simulink model "gm_sampleModel1471_5_sub"  (R2023a)
settings: Solver=VariableStepAuto  StartTime=0.0  StopTime=10.0  RelTol=1e-3
libraries: simulink x5, hdlsllib x1
settings Model: Creator=user1  LastModifiedBy=user1
settings OptimizationCC: BlockReduction=off  ConditionallyExecuteInputs=off
settings DebuggingCC: InheritedTsInSrcMsg=none

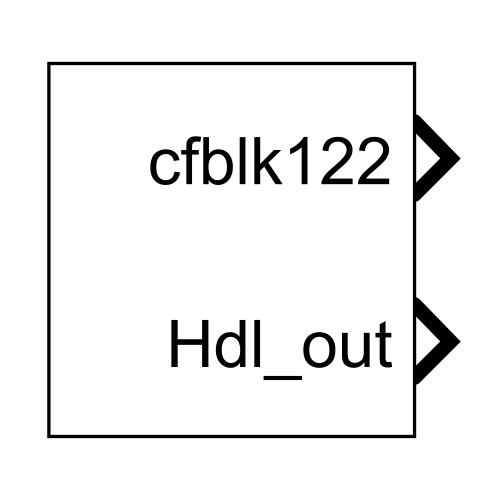
[thumbnail: Simulink's stored preview of the top-level diagram]
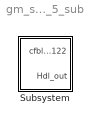
== system gm_sampleModel1471_5_sub ==
  Subsystem : Subsystem

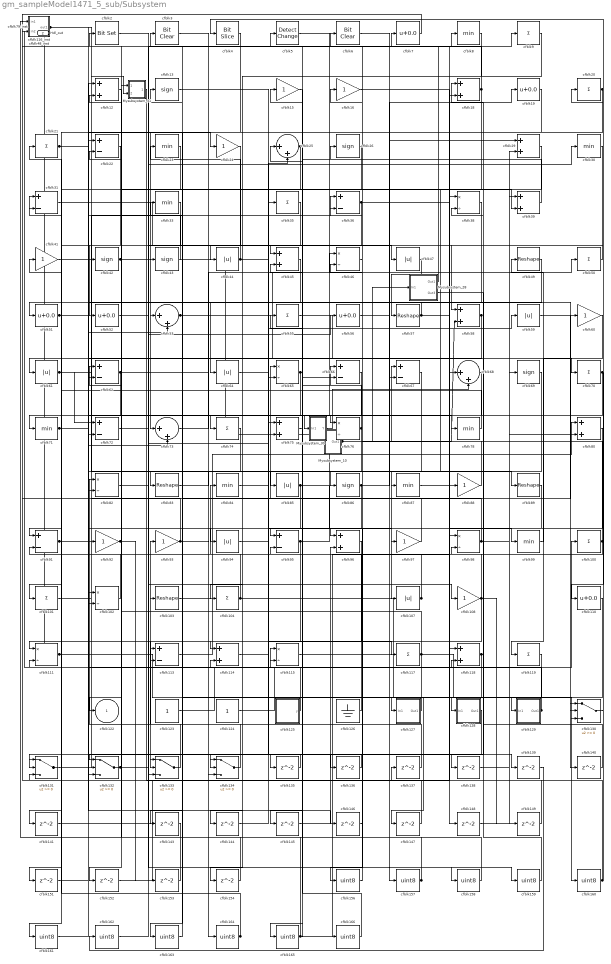
== system gm_sampleModel1471_5_sub/Subsystem ==
  Mysubsystem_10 : Subsystem
  Mysubsystem_28 : Subsystem
  Mysubsystem_30 : Subsystem
  Mysubsystem_31 : Subsystem
  cfblk{9,20..21,35,50,55,70,74,100..101,104,117,119} (13 alike) : Sum  Inputs=+  OutDataTypeStr=uint8
  cfblk{38,46,65,76,82,98,102,111,115} (9 alike) : Product  Inputs=*/  OutDataTypeStr=uint8  RndMeth=Zero  SaturateOnIntegerOverflow=on
  cfblk{49,57,83,89,103} (5 alike) : Reshape
  cfblk{44,47,59,61,64,85,94,107} (8 alike) : Abs  OutDataTypeStr=uint8  SaturateOnIntegerOverflow=off
  cfblk{15..16,24,41,60,88,92..93,97,108} (10 alike) : Gain  OutDataTypeStr=uint8
  cfblk{7,19,51..52,56,110} (6 alike) : Bias  Bias=0.0  SaturateOnIntegerOverflow=off
  cfblk{22,31,36,62,66..67,72,91,95,113} (10 alike) : Sum  Inputs=+-  OutDataTypeStr=uint8
  cfblk{12,18,29,39,45,58,75,80,96,114,118} (11 alike) : Sum  OutDataTypeStr=uint8
  cfblk116_inst : Subsystem
  cfblk123 : Constant  OutDataTypeStr=uint8  SampleTime=-1
  cfblk124 : Constant  OutDataTypeStr=uint8  SampleTime=-1
  cfblk125 : Subsystem  mask(Counter Free-Running){NumBits=double(16), tsamp=double(-1)}
      mask prompts: NumBits "Simulink:masks:NumberOfBits_MP"; tsamp "Simulink:masks:SampleTime_MP"
      mask help: Simulink:masks:CounterFreeRunning_MD
  cfblk126 : Ground
  cfblk127 : Subsystem
  cfblk128 : Subsystem
  cfblk129 : Subsystem
  cfblk{13,26,42..43,69,86} (6 alike) : Signum
  cfblk{130..134} (5 alike) : Switch  OutDataTypeStr=uint8  SaturateOnIntegerOverflow=off  InputSameDT=off
  cfblk{135..141,143..149,151..154} (18 alike) : Delay  SampleTime=1
  cfblk{156..166} (11 alike) : DataTypeConversion  OutDataTypeStr=uint8  SaturateOnIntegerOverflow=off  RndMeth=Floor
  cfblk2 : simulink/Logic and Bit Operations/Bit Set  iBit=0
      settings: LibrarySourceBlock=|
      | hdlsllib/Logic and Bit
      | Operations/Bit Set
  cfblk{8,23,30,33,71,78,84,87,99} (9 alike) : MinMax  OutDataTypeStr=uint8
  cfblk{25,53,68,73} (4 alike) : Sum  Inputs=|++  OutDataTypeStr=uint8
  cfblk3 : simulink/Logic and Bit Operations/Bit Clear  iBit=0
      settings: LibrarySourceBlock=|
      | hdlsllib/Logic and Bit
      | Operations/Bit Clear
  cfblk4 : hdlsllib/Logic and Bit Operations/Bit Slice  lidx=7  ridx=0
  cfblk48_inst : Subsystem
  cfblk5 : simulink/Logic and Bit Operations/Detect Change  vinit=0  OutDataTypeStr=uint8
      settings: LibrarySourceBlock=|
      | hdlsllib/Logic and Bit
      | Operations/Detect
      | Change
  cfblk6 : simulink/Logic and Bit Operations/Bit Clear  iBit=0
      settings: LibrarySourceBlock=|
      | hdlsllib/Logic and Bit
      | Operations/Bit Clear
  cfblk79_inst : Subsystem
  cfblk122 : Outport  OutDataTypeStr=uint8  SampleTime=1  VectorParamsAs1DForOutWhenUnconnected=off
  Hdl_out : Outport  Port=2  OutDataTypeStr=uint8  SampleTime=1
  wires:
  Mysubsystem_10/1(Out1) -> cfblk58/2, Mysubsystem_28/1(In1)
  Mysubsystem_28/1(Out1) -> cfblk7/1
  Mysubsystem_28/2(Out3) -> cfblk133/2
  Mysubsystem_30/1(Y) -> cfblk68/2
  Mysubsystem_31/1(Out1) -> cfblk137/1
  cfblk100/1 -> cfblk91/2, cfblk67/1
  cfblk101/1 -> cfblk36/1
  cfblk102/1 -> cfblk82/1
  cfblk103/1 -> cfblk80/1
  cfblk104/1 -> cfblk128/1(In1), cfblk84/1
  cfblk107/1 -> cfblk95/2, cfblk26/1
  cfblk108/1 -> cfblk36/2, cfblk133/1, cfblk149/1
  cfblk110/1 -> cfblk127/1(In1)
  cfblk111/1 -> Hdl_out/1, cfblk129/1(In1)
  cfblk113/1 -> cfblk65/1
  cfblk114/1 -> cfblk35/1
  cfblk115/1 -> cfblk160/1
  cfblk116_inst/1(out1) -> cfblk107/1, Mysubsystem_31/2(In2)
  cfblk117/1 -> cfblk22/2, cfblk130/3, cfblk114/2
  cfblk118/1 -> cfblk18/1, cfblk147/1
  cfblk119/1 -> cfblk163/1
  cfblk12/1 -> cfblk39/2
  cfblk123/1 -> cfblk18/2
  cfblk124/1 -> cfblk100/1
  cfblk125/1(y) -> cfblk62/1
  cfblk126/1 -> cfblk12/2
  cfblk127/1(Out1) -> cfblk46/2
  cfblk128/1(Out1) -> cfblk135/1
  cfblk129/1(Out1) -> cfblk79_inst/2(in2), cfblk45/2, cfblk25/1
  cfblk13/1 -> cfblk75/2
  cfblk130/1 -> cfblk4/1
  cfblk131/1 -> cfblk60/1
  cfblk132/1 -> cfblk75/1, cfblk8/1
  cfblk133/1 -> cfblk92/1
  cfblk134/1 -> cfblk93/1
  cfblk135/1 -> cfblk131/2
  cfblk136/1 -> cfblk134/2
  cfblk137/1 -> cfblk102/1
  cfblk138/1 -> cfblk39/1
  cfblk139/1 -> cfblk162/1
  cfblk140/1 -> cfblk118/2
  cfblk141/1 -> cfblk68/1
  cfblk143/1 -> cfblk116_inst/1(in1)
  cfblk144/1 -> cfblk65/2
  cfblk145/1 -> cfblk96/2
  cfblk146/1 -> cfblk66/1
  cfblk147/1 -> cfblk131/3
  cfblk148/1 -> cfblk80/2
  cfblk149/1 -> cfblk113/2
  cfblk15/1 -> cfblk165/1
  cfblk151/1 -> cfblk82/2
  cfblk152/1 -> cfblk25/2
  cfblk153/1 -> cfblk111/2
  cfblk154/1 -> cfblk22/1
  cfblk156/1 -> cfblk6/1
  cfblk157/1 -> cfblk31/1, cfblk41/1
  cfblk158/1 -> cfblk2/1
  cfblk159/1 -> cfblk98/2
  cfblk16/1 -> cfblk99/1
  cfblk160/1 -> cfblk48_inst/2(in2), cfblk38/2, cfblk20/1
  cfblk161/1 -> cfblk115/1
  cfblk162/1 -> cfblk115/2
  cfblk163/1 -> cfblk3/1
  cfblk164/1 -> cfblk31/2, cfblk103/1
  cfblk165/1 -> cfblk13/1, cfblk98/1
  cfblk166/1 -> cfblk15/1
  cfblk18/1 -> cfblk79_inst/1(in1), cfblk134/3
  cfblk19/1 -> cfblk143/1
  cfblk2/1 -> cfblk159/1
  cfblk20/1 -> cfblk73/1, cfblk51/1
  cfblk21/1 -> cfblk67/2, cfblk53/1
  cfblk22/1 -> cfblk91/1
  cfblk23/1 -> cfblk132/1
  cfblk24/1 -> cfblk132/3
  cfblk25/1 -> cfblk61/1, cfblk131/1
  cfblk26/1 -> cfblk145/1
  cfblk29/1 -> cfblk87/1
  cfblk3/1 -> cfblk164/1
  cfblk30/1 -> cfblk58/1
  cfblk31/1 -> cfblk47/1
  cfblk33/1 -> cfblk52/1
  cfblk35/1 -> cfblk83/1
  cfblk36/1 -> cfblk148/1, cfblk104/1
  cfblk38/1 -> cfblk144/1
  cfblk39/1 -> cfblk5/1
  cfblk4/1 -> cfblk43/1
  cfblk41/1 -> cfblk130/2
  cfblk42/1 -> cfblk44/1, cfblk76/2
  cfblk43/1 -> cfblk12/1
  cfblk44/1 -> cfblk96/1, cfblk23/1
  cfblk45/1 -> cfblk64/1
  cfblk46/1 -> cfblk16/1
  cfblk47/1 -> cfblk57/1
  cfblk48_inst/1(out1) -> cfblk53/2
  cfblk49/1 -> cfblk141/1
  cfblk5/1 -> cfblk118/1
  cfblk50/1 -> cfblk45/1
  cfblk51/1 -> cfblk139/1, cfblk78/1
  cfblk52/1 -> cfblk30/1
  cfblk53/1 -> cfblk29/2, cfblk140/1
  cfblk55/1 -> cfblk70/1
  cfblk56/1 -> cfblk158/1
  cfblk57/1 -> Mysubsystem_31/1(In1), cfblk9/1
  cfblk58/1 -> cfblk151/1, cfblk101/1
  cfblk59/1 -> cfblk130/1
  cfblk6/1 -> cfblk157/1
  cfblk60/1 -> cfblk119/1
  cfblk61/1 -> cfblk89/1, cfblk72/1
  cfblk62/1 -> cfblk72/2, Mysubsystem_30/1(In1)
  cfblk64/1 -> cfblk138/1
  cfblk65/1 -> cfblk94/1, cfblk166/1
  cfblk66/1 -> cfblk71/1
  cfblk67/1 -> cfblk114/1
  cfblk68/1 -> cfblk85/1
  cfblk69/1 -> cfblk152/1
  cfblk7/1 -> cfblk48_inst/1(in1)
  cfblk70/1 -> cfblk110/1, cfblk74/1
  cfblk71/1 -> cfblk73/2, cfblk146/1
  cfblk72/1 -> cfblk56/1
  cfblk73/1 -> cfblk50/1
  cfblk74/1 -> cfblk132/2
  cfblk75/1 -> cfblk66/2
  cfblk76/1 -> cfblk95/1, cfblk55/1
  cfblk78/1 -> cfblk21/1
  cfblk79_inst/1(out1) -> cfblk24/1
  cfblk8/1 -> cfblk134/1
  cfblk80/1 -> cfblk102/2
  cfblk82/1 -> cfblk108/1
  cfblk83/1 -> cfblk86/1
  cfblk84/1 -> cfblk59/1
  cfblk85/1 -> cfblk113/1, cfblk97/1
  cfblk86/1 -> cfblk29/1, cfblk19/1, cfblk122/1
  cfblk87/1 -> cfblk88/1
  cfblk88/1 -> cfblk46/1
  cfblk89/1 -> cfblk156/1
  cfblk9/1 -> cfblk154/1
  cfblk91/1 -> cfblk42/1, cfblk133/3
  cfblk92/1 -> cfblk62/2, cfblk153/1
  cfblk93/1 -> cfblk116_inst/2(in2), cfblk136/1
  cfblk94/1 -> cfblk117/1
  cfblk95/1 -> cfblk161/1, cfblk38/1
  cfblk96/1 -> cfblk111/1
  cfblk97/1 -> cfblk76/1
  cfblk98/1 -> cfblk69/1, cfblk33/1
  cfblk99/1 -> cfblk49/1

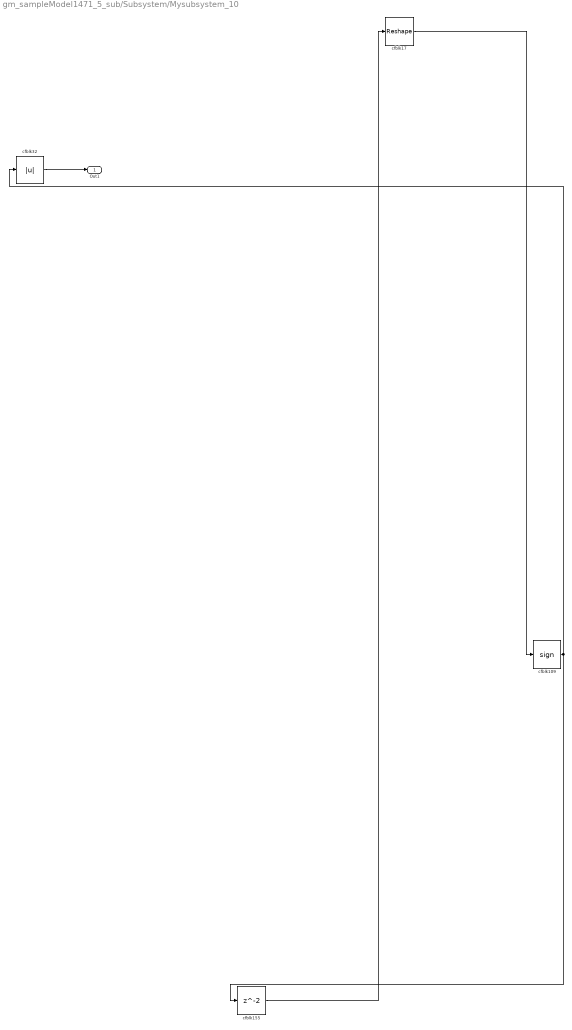
== system gm_sampleModel1471_5_sub/Subsystem/Mysubsystem_10 ==
  cfblk109 : Signum
  cfblk155 : Delay  SampleTime=1
  cfblk17 : Reshape
  cfblk32 : Abs  SaturateOnIntegerOverflow=off
  Out1 : Outport  SampleTime=1
  wires:
  cfblk109/1 -> cfblk32/1, cfblk155/1
  cfblk155/1 -> cfblk17/1
  cfblk17/1 -> cfblk109/1
  cfblk32/1 -> Out1/1

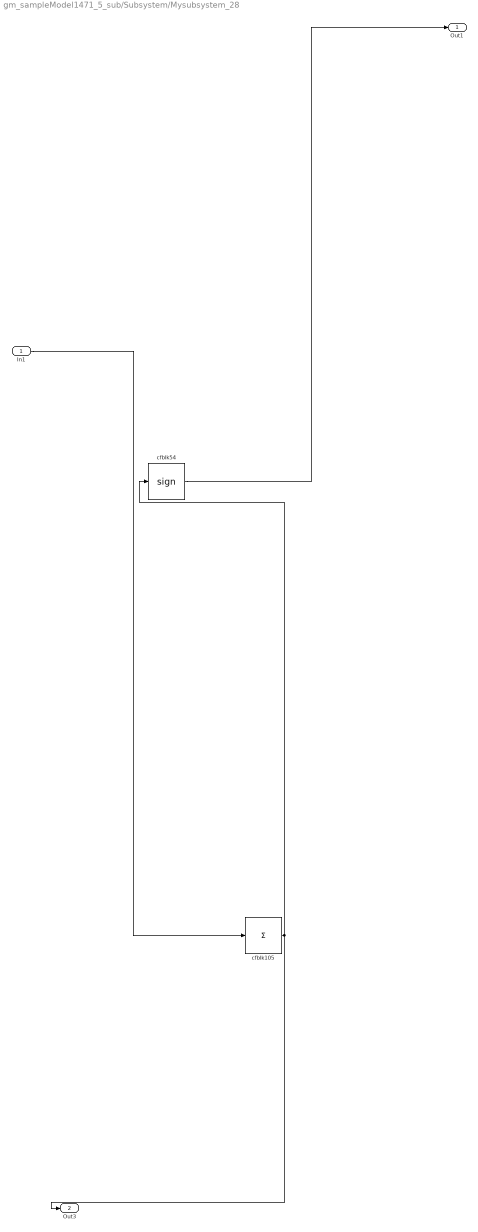
== system gm_sampleModel1471_5_sub/Subsystem/Mysubsystem_28 ==
  In1 : Inport  OutDataTypeStr=uint8  PortDimensions=1  SampleTime=1
  cfblk105 : Sum  Inputs=+
  cfblk54 : Signum
  Out1 : Outport  SampleTime=1
  Out3 : Outport  Port=2  SampleTime=1
  wires:
  In1/1 -> cfblk105/1
  cfblk105/1 -> cfblk54/1, Out3/1
  cfblk54/1 -> Out1/1

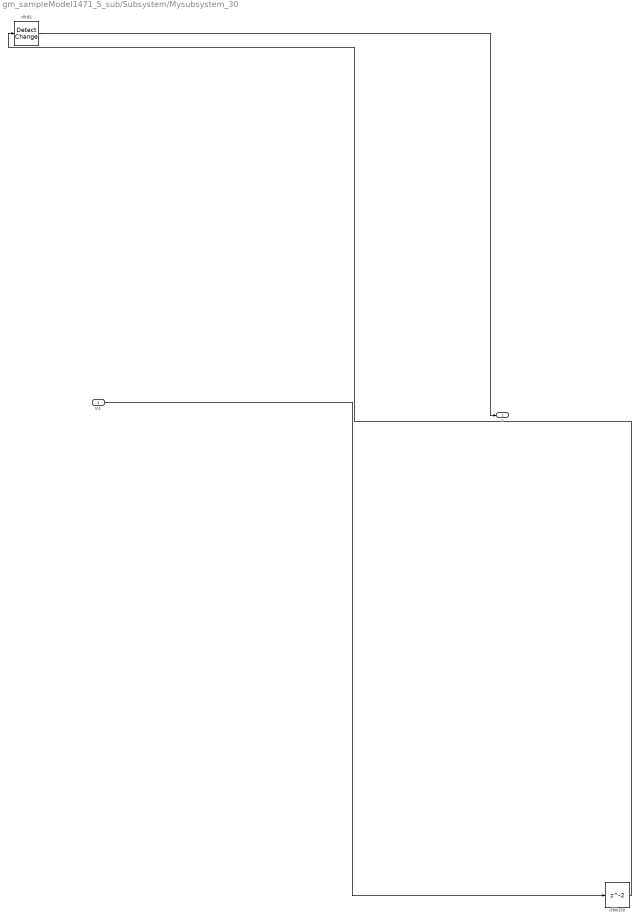
== system gm_sampleModel1471_5_sub/Subsystem/Mysubsystem_30 ==
  In1 : Inport  OutDataTypeStr=uint8  PortDimensions=1  SampleTime=1
  cfblk1 : simulink/Logic and Bit Operations/Detect Change  vinit=0  OutDataTypeStr=boolean
      settings: LibrarySourceBlock=|
      | hdlsllib/Logic and Bit
      | Operations/Detect
      | Change
  cfblk150 : Delay  SampleTime=1
  Y : Outport  SampleTime=1
  wires:
  In1/1 -> cfblk150/1
  cfblk1/1 -> Y/1
  cfblk150/1 -> cfblk1/1

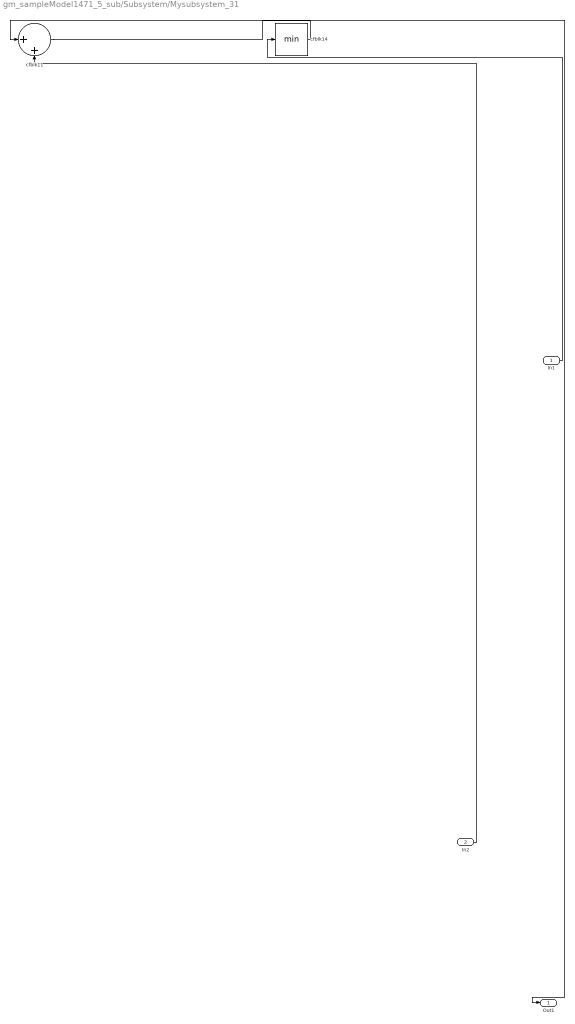
== system gm_sampleModel1471_5_sub/Subsystem/Mysubsystem_31 ==
  In1 : Inport  OutDataTypeStr=uint8  PortDimensions=1  SampleTime=1
  In2 : Inport  Port=2  OutDataTypeStr=uint8  PortDimensions=1  SampleTime=1
  cfblk11 : Sum  Inputs=|++
  cfblk14 : MinMax
  Out1 : Outport  SampleTime=1
  wires:
  In1/1 -> cfblk14/1
  In2/1 -> cfblk11/2
  cfblk11/1 -> Out1/1
  cfblk14/1 -> cfblk11/1

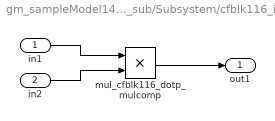
== system gm_sampleModel1471_5_sub/Subsystem/cfblk116_inst ==
  in1 : Inport  OutDataTypeStr=uint8  SampleTime=1
  in2 : Inport  Port=2  OutDataTypeStr=uint8  SampleTime=1
  mul_cfblk116_dotp_mulcomp : Product  Inputs=**  OutDataTypeStr=uint8  SampleTime=1
  out1 : Outport  OutDataTypeStr=uint8  SampleTime=1
  wires:
  in1/1 -> mul_cfblk116_dotp_mulcomp/1
  in2/1 -> mul_cfblk116_dotp_mulcomp/2
  mul_cfblk116_dotp_mulcomp/1 -> out1/1

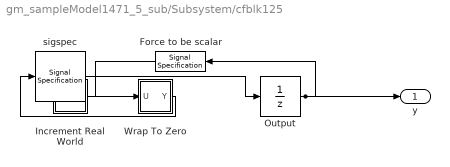
== system gm_sampleModel1471_5_sub/Subsystem/cfblk125 ==
  Force to be scalar : SignalSpecification  DisableCoverage=on  Dimensions=1
  Increment Real World : Subsystem  mask(Real World Value Increment){}
      mask help: Simulink:masks:RealWorldValueIncrement_MD
      mask Display: disp('V++')
  Output : UnitDelay  InitialCondition=0.0  SampleTime=tsamp  HasFrameUpgradeWarning=on
  Wrap To Zero : Subsystem  mask(Wrap To Zero){Threshold=double(65535)}
      mask prompts: Threshold "Simulink:masks:Threshold_MP"
      mask help: Simulink:masks:WrapToZero_MD
  sigspec : SignalSpecification  OutDataTypeStr=uint16  Dimensions=1
  y : Outport  SampleTime=1
  wires:
  Force to be scalar/1 -> Increment Real World/1(u)
  Increment Real World/1(y) -> Wrap To Zero/1(U)
  Output/1 -> Force to be scalar/1, y/1
  Wrap To Zero/1(Y) -> sigspec/1
  sigspec/1 -> Output/1

== system gm_sampleModel1471_5_sub/Subsystem/cfblk127 ==
  In1 : Inport  OutDataTypeStr=uint8  PortDimensions=1  SampleTime=1
  Out1 : Outport  SampleTime=1
  wires:
  In1/1 -> Out1/1

== system gm_sampleModel1471_5_sub/Subsystem/cfblk128 ==
  In1 : Inport  OutDataTypeStr=uint8  PortDimensions=1  SampleTime=1
  Out1 : Outport  SampleTime=1
  wires:
  In1/1 -> Out1/1

== system gm_sampleModel1471_5_sub/Subsystem/cfblk129 ==
  In1 : Inport  OutDataTypeStr=uint8  PortDimensions=1  SampleTime=1
  Out1 : Outport  SampleTime=1
  wires:
  In1/1 -> Out1/1

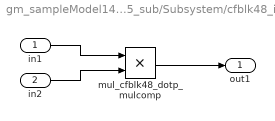
== system gm_sampleModel1471_5_sub/Subsystem/cfblk48_inst ==
  in1 : Inport  OutDataTypeStr=uint8  SampleTime=1
  in2 : Inport  Port=2  OutDataTypeStr=uint8  SampleTime=1
  mul_cfblk48_dotp_mulcomp : Product  Inputs=**  OutDataTypeStr=uint8  SampleTime=1
  out1 : Outport  OutDataTypeStr=uint8  SampleTime=1
  wires:
  in1/1 -> mul_cfblk48_dotp_mulcomp/1
  in2/1 -> mul_cfblk48_dotp_mulcomp/2
  mul_cfblk48_dotp_mulcomp/1 -> out1/1

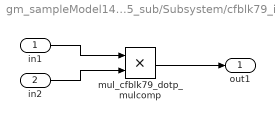
== system gm_sampleModel1471_5_sub/Subsystem/cfblk79_inst ==
  in1 : Inport  OutDataTypeStr=uint8  SampleTime=1
  in2 : Inport  Port=2  OutDataTypeStr=uint8  SampleTime=1
  mul_cfblk79_dotp_mulcomp : Product  Inputs=**  OutDataTypeStr=uint8  SampleTime=1
  out1 : Outport  OutDataTypeStr=uint8  SampleTime=1
  wires:
  in1/1 -> mul_cfblk79_dotp_mulcomp/1
  in2/1 -> mul_cfblk79_dotp_mulcomp/2
  mul_cfblk79_dotp_mulcomp/1 -> out1/1

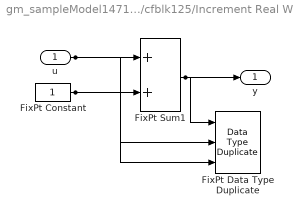
== system gm_sampleModel1471_5_sub/Subsystem/cfblk125/Increment Real World ==
  u : Inport  OutDataTypeStr=uint16  SampleTime=1
  FixPt Constant : Constant  DisableCoverage=on  OutDataTypeStr=Inherit: Inherit via back propagation  SampleTime=-1
  FixPt Data Type Duplicate : DataTypeDuplicate  DisableCoverage=on  NumInputPorts=3
  FixPt Sum1 : Sum  InputSameDT=on  OutDataTypeStr=Inherit: Inherit via back propagation  LockScale=on
  y : Outport  SampleTime=1
  wires:
  u/1 -> FixPt Sum1/1, FixPt Data Type Duplicate/2
  FixPt Constant/1 -> FixPt Sum1/2, FixPt Data Type Duplicate/3
  FixPt Sum1/1 -> FixPt Data Type Duplicate/1, y/1

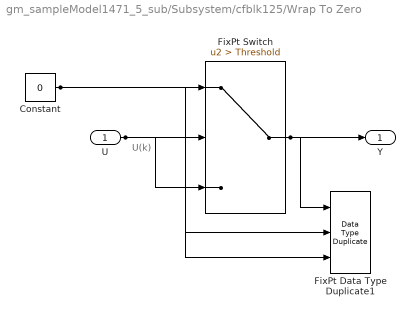
== system gm_sampleModel1471_5_sub/Subsystem/cfblk125/Wrap To Zero ==
  note: U(k)
  U : Inport  OutDataTypeStr=uint16  SampleTime=1
  Constant : Constant  DisableCoverage=on  Value=0  OutDataTypeStr=Inherit: Inherit via back propagation  SampleTime=-1
  FixPt Data Type Duplicate1 : DataTypeDuplicate  DisableCoverage=on  NumInputPorts=3
  FixPt Switch : Switch  Criteria=u2 > Threshold  Threshold=Threshold  OutDataTypeStr=Inherit: Inherit via back propagation  ZeroCross=off  SaturateOnIntegerOverflow=off  InputSameDT=off
  Y : Outport  SampleTime=1
  wires:
  U/1 -> FixPt Switch/3, FixPt Switch/2, FixPt Data Type Duplicate1/2
  Constant/1 -> FixPt Switch/1, FixPt Data Type Duplicate1/3
  FixPt Switch/1 -> FixPt Data Type Duplicate1/1, Y/1
